simulink model "xlink"  (Simulink 6.6)
settings: Solver=ode45  StartTime=0.0  StopTime=10.0  RelTol=1e-3
settings Model: Creator=cox  LastModifiedBy=cox  ExtModeAutoUpdateStatusClock=off

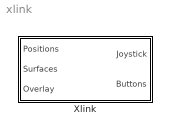
== system xlink ==
  Xlink : Subsystem  mask(Xlink){HUDCell={'alpha','beta','Velocity'}}
      mask prompts: HUDCell "Lables for HUD, (cell array)"
      mask help:
      | Input Positions and Surfaces for X-Plane Visualization.
      |   Positions - [ Latitude, Longitude, Altitude, Roll, Pitch, Yaw] % degrees and ft.
      |   Surfaces  - [ Aileron, Elevator, Rudder, Flaps, Spoiler, GearDown] % deg and 0/1
      |
      | Output is Joysick axes and Button pushes.
      |   Joystick - First 16 axes
      |   Buttons  - 16 buttons as assigned to Xlink in X-Plane
      mask init:
      | if isempty(HUDCell) HUDCell=cell(6,1); end
      | HUDTextArray = uint8(zeros(90,1));
      | 
      | % loop through names, assign to string arrays
      | for i=1:min(length(HUDCell),6);
      |   if length(HUDCell{i})>14 HUDCell{i}=HUDCell{i}(1:14); end
      |   if length(HUDCell{i}>0),
      |     HUDTextArray((i-1)*15+1:(i-1)*15+length(HUDCell{i})) = uint8(HUDCell{i});
      |   end
      | end

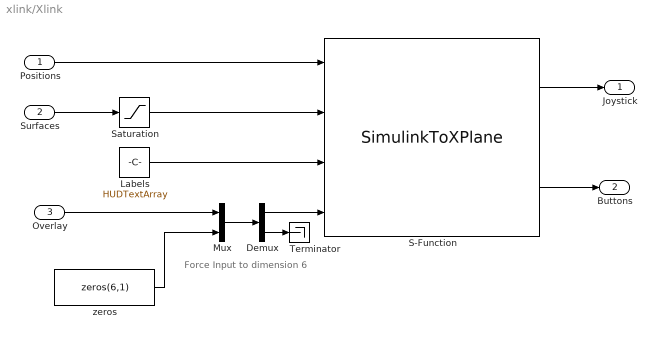
== system xlink/Xlink ==
  note: Force Input to
      | dimension 6
  Positions : Inport
  Surfaces : Inport  Port=2
  Overlay : Inport  Port=3
  Demux : Demux  Outputs=[6 -1]
  Labels : Constant  Value=HUDTextArray  OutDataTypeMode=uint8
  Mux : Mux  Inputs=2
  S-Function : S-Function  FunctionName=SimulinkToXPlane
  Saturation : Saturate  UpperLimit=[180*ones(5,1); 1]  LowerLimit=[-180*ones(5,1); 0]
  Terminator : Terminator
  zeros : Constant  Value=zeros(6,1)  OutDataTypeMode=double
  Joystick : Outport
  Buttons : Outport  Port=2
  wires:
  Positions/1 -> S-Function/1
  S-Function/1 -> Joystick/1
  Surfaces/1 -> Saturation/1
  S-Function/2 -> Buttons/1
  Saturation/1 -> S-Function/2
  Labels/1 -> S-Function/3
  Overlay/1 -> Mux/1
  zeros/1 -> Mux/2
  Mux/1 -> Demux/1
  Demux/1 -> S-Function/4
  Demux/2 -> Terminator/1
